simulink model "model_stribeck"  (R2023a)
settings: Solver=ode45  StartTime=0.0  StopTime=4  FixedStep=dt  MaxStep=0.001  RelTol=1e-3
values from neighbouring files (symbols this model uses):
  IC = [0.06 3.14159265359 0 0]    [WYNIKI2.mat]    (also in ogladanieWynikow.m = x0low; program_main.m = x0low)
settings Model: Creator=Adam  LastModifiedBy=Adam
settings SolverCC: AlgebraicLoopSolver=TrustRegion
settings DataIOCC: ExternalInput=ind  LoadExternalInput=on  SignalLogging=off  DSMLogging=off  OutputSaveName=out  ReturnWorkspaceOutputsName=sout
settings OptimizationCC: SimCompilerOptimization=on  AccelVerboseBuild=on
settings DebuggingCC: AlgebraicLoopMsg=none  UnconnectedInputMsg=warning  UnconnectedOutputMsg=warning  UnconnectedLineMsg=warning
settings ModelReferenceCC: EnableRefExpFcnMdlSchedulingChecks=on
settings RTWCC: DLArmComputeVersion=19.05

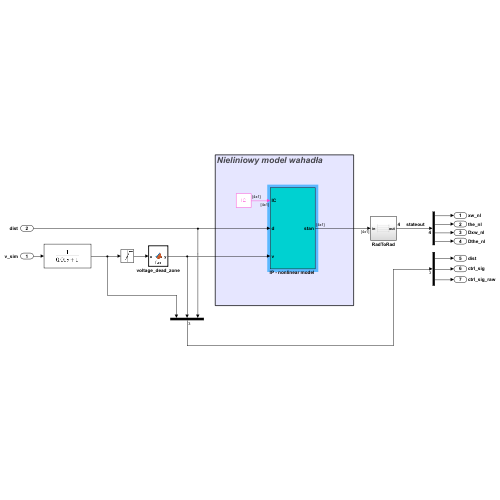
[thumbnail: Simulink's stored preview of the top-level diagram]
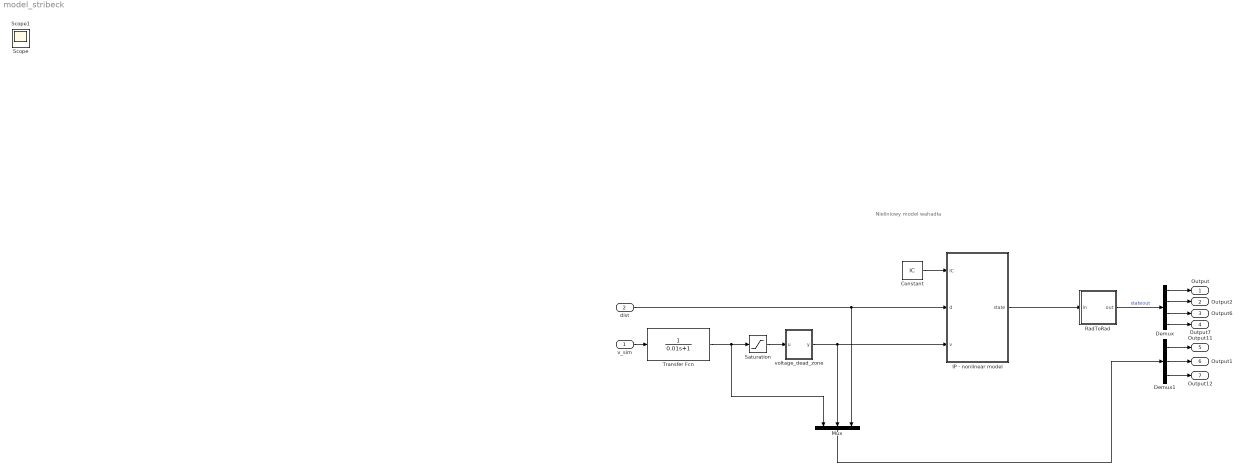
== system model_stribeck ==
  note: Nieliniowy model wahadła
  v_sim : Inport
  dist : Inport  Port=2
  Constant : Constant  Value=IC  VectorParams1D=off
  Demux : Demux
  Demux1 : Demux  Outputs=3
  "IP - nonlinear model " : Subsystem  Description=Nonlinear model of inverted pendulum
      mask Display:
      | port_label('output', 1, 'stan');
      | port_label('input', 1, 'IC');
      | port_label('input', 2, 'd');
      | port_label('input', 3, 'v');
  Mux : Mux  Inputs=3
  RadToRad : Subsystem
  Saturation : Saturate  UpperLimit=12  LowerLimit=-12
  Transfer Fcn : TransferFcn  Denominator=[0.01 1]
  voltage_dead_zone : MATLAB Function  TreatAsAtomicUnit=on
  Output : Outport  SignalName=xw_nl
  Output2 : Outport  Port=2  SignalName=the_nl
  Output6 : Outport  Port=3  SignalName=Dxw_nl
  Output7 : Outport  Port=4  SignalName=Dthe_nl
  Output11 : Outport  Port=5  SignalName=dist
  Output1 : Outport  Port=6  SignalName=ctrl_sig
  Output12 : Outport  Port=7  SignalName=ctrl_sig_raw
  Scope : Scope
  Scope1 : Scope
  wires:
  "IP - nonlinear model "/1(state) -> RadToRad/1(in)
  Constant/1 -> "IP - nonlinear model "/1(IC)
  dist/1 -> Mux/3, "IP - nonlinear model "/2(d)
  RadToRad/1(out) -> Demux/1  "stateout"
  Demux/1 -> Output/1
  Demux/2 -> Output2/1
  Demux/3 -> Output6/1
  Demux/4 -> Output7/1
  Mux/1 -> Demux1/1
  Demux1/1 -> Output11/1
  Demux1/2 -> Output1/1
  Demux1/3 -> Output12/1
  Saturation/1 -> voltage_dead_zone/1(u)
  voltage_dead_zone/1(y) -> Mux/2, "IP - nonlinear model "/3(v)
  v_sim/1 -> Transfer Fcn/1
  Transfer Fcn/1 -> Mux/1, Saturation/1

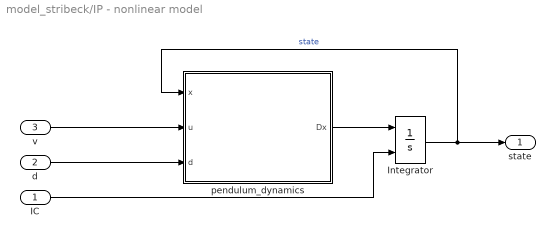
== system model_stribeck/IP - nonlinear model  ==
  IC : Inport
  d : Inport  Port=2
  v : Inport  Port=3
  Integrator : Integrator  InitialConditionSource=external
  pendulum_dynamics : MATLAB Function  TreatAsAtomicUnit=on
  state : Outport
  wires:
  Integrator/1 -> state/1, pendulum_dynamics/1(x)  "state"
  v/1 -> pendulum_dynamics/2(u)
  pendulum_dynamics/1(Dx) -> Integrator/1
  IC/1 -> Integrator/2
  d/1 -> pendulum_dynamics/3(d)

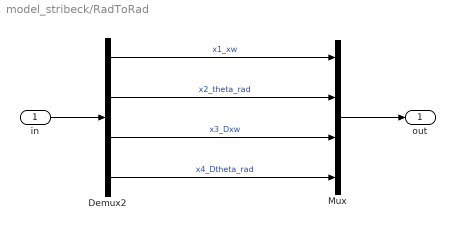
== system model_stribeck/RadToRad ==
  in : Inport
  Demux2 : Demux
  Mux : Mux
  out : Outport
  wires:
  Demux2/1 -> Mux/1  "x1_xw"
  Demux2/2 -> Mux/2  "x2_theta_rad"
  in/1 -> Demux2/1
  Demux2/3 -> Mux/3  "x3_Dxw"
  Demux2/4 -> Mux/4  "x4_Dtheta_rad"
  Mux/1 -> out/1

== matlab function model_stribeck/voltage_dead_zone ==
  data: u input; y output; dead_zone_ampl parameter
function y = fcn(u, dead_zone_ampl)
    if (abs(u) < dead_zone_ampl)
        y = 0;
    else
        y = u;
    end
end

== matlab function model_stribeck/IP - nonlinear model /pendulum_dynamics ==
  data: x input; u input; d input; Dx output; params_stribeck parameter
function Dx = dynamika_wahadla(x, u, d, params_stribeck)
% x : stan
% u : input - napięcie
%
% params scope: "parameters"
%

% State, function input: x = [x Dx theta Dtheta]'
% x1 = x(1);
x2 = x(2);
x3 = x(3);
x4 = x(4);

params_stribeck = num2cell(params_stribeck);
[alpha_dcm, beta_dcm, b_stri, gamma_stri, miu_c, miu_s, vs, M, mp, mc, Lp] = params_stribeck{:};

g = 9.8145;
Lc = 2*Lp;
mr = mc + mp;
Mt = mr + M;
L = (Lc*mc + Lp*mp) / mr;
Jcm = 0.3333333*mp*Lp^2 + mp*(L-Lp)^2 + mc*(L-Lc)^2;
Jt = Jcm + mr*L^2;

i_i = 2;
delta_ = 600;

Ff = (miu_c + (miu_s-miu_c)*exp(-(x3/vs)^i_i)) * Mt*g*tanh(delta_*x3) + b_stri*x3;
Fi = alpha_dcm*u - beta_dcm*x3;
A = d*cos(x2) - Ff + L*mr*x4^2*sin(x2) + Fi;
B = d*Lc + L*g*mr*sin(x2) - gamma_stri*x4;
DEN = Jt*Mt - (L*mr*cos(x2))^2;

ddt_x1 = x3;
ddt_x2 = x4;
ddt_x3 = (Jt*A - L*mr*cos(x2)*B) / DEN;
ddt_x4 = (Mt*B - L*mr*cos(x2)*A) / DEN;

% output
Dx = [ddt_x1 ddt_x2 ddt_x3 ddt_x4]';

end
